simulink model "SimBG"  (R2023b)
settings: Solver=VariableStepAuto  StartTime=0.0  StopTime=t_sim  MaxStep=1e-2  RelTol=1e-3
values from neighbouring files (symbols this model uses):
  BG_0 = 120    [Batch_test_Cryer.m]    (also in Step_test.m; example_batch_testing.m; glucagon_dependency_test.m; init.m)
  control_flag = false    [Batch_test_Cryer.m]    (also in example_batch_testing.m; glucagon_dependency_test.m; init.m)
  G_GNG = 6    [Batch_test_Cryer.m]    (also in example_batch_testing.m; glucagon_dependency_test.m; init.m)
  glucagon_dose = 1e7    (= 10000000)    [Batch_test_Cryer.m]    (also in example_batch_testing.m; glucagon_dependency_test.m; init.m)
  Hyper_Hyst_H = (Hyper_Threshold + 10)/18    (= 10.5555555556)    [Batch_test_Cryer.m]    (also in example_batch_testing.m; glucagon_dependency_test.m; init.m)
  Hyper_Hyst_L = (Hyper_Threshold - 10)/18    (= 9.44444444444)    [Batch_test_Cryer.m]    (also in example_batch_testing.m; glucagon_dependency_test.m; init.m)
  Hyper_Threshold = 180    [Batch_test_Cryer.m]    (also in example_batch_testing.m; glucagon_dependency_test.m; init.m)
  Hypo_Hyst_H = (Hypo_Threshold+10)/18    (= 4.44444444444)    [Batch_test_Cryer.m]    (also in example_batch_testing.m; glucagon_dependency_test.m; init.m)
  Hypo_Hyst_L = (Hypo_Threshold-10)/18    (= 3.33333333333)    [Batch_test_Cryer.m]    (also in example_batch_testing.m; glucagon_dependency_test.m; init.m)
  Hypo_Threshold = 70    [Batch_test_Cryer.m]    (also in example_batch_testing.m; glucagon_dependency_test.m; init.m)
  k_bi = rand*0.05+0.075    [Batch_test_Cryer.m]    (also in example_batch_testing.m; init.m)
  K_d_glu = 2.484    [Batch_test_Cryer.m]    (also in example_batch_testing.m; glucagon_dependency_test.m; init.m = 1)
  K_d_ins = 379.0122/ICR -5.8677    [Batch_test_Cryer.m]    (also in example_batch_testing.m; glucagon_dependency_test.m; init.m)
  K_i_glu = 0    [Batch_test_Cryer.m]    (also in example_batch_testing.m; glucagon_dependency_test.m; init.m)
  K_i_ins = 0    [Batch_test_Cryer.m]    (also in example_batch_testing.m; glucagon_dependency_test.m; init.m)
  K_p_glu = 0.10976    [Batch_test_Cryer.m]    (also in example_batch_testing.m; glucagon_dependency_test.m; init.m = 0.1)
  K_p_ins = 0.1    [Batch_test_Cryer.m]    (also in example_batch_testing.m; glucagon_dependency_test.m; init.m)
  M_g = 180.16    [Batch_test_Cryer.m]    (also in example_batch_testing.m; glucagon_dependency_test.m; init.m)
  sig_n = 10    [Batch_test_Cryer.m]    (also in example_batch_testing.m; glucagon_dependency_test.m; init.m)
  T_CGM = 5    [Batch_test_Cryer.m]    (also in example_batch_testing.m; glucagon_dependency_test.m; init.m)
  T_CTRL = 5    [Batch_test_Cryer.m]    (also in example_batch_testing.m; glucagon_dependency_test.m; init.m)
  t_sim = minutes(end_time - start_time)    [Batch_test_Cryer.m]    (also in Step_test.m = 1800; example_batch_testing.m; glucagon_dependency_test.m; init.m = 1800)
  TDD_limit = 0.6*W*1000    (= 42000)    [Batch_test_Cryer.m]    (also in example_batch_testing.m; glucagon_dependency_test.m; init.m)
  U_b0 = fzero(f, 10)    [Batch_test_Cryer.m]    (also in Step_test.m; cohort_generation.m; example_batch_testing.m; glucagon_dependency_test.m)
  W = 70    [Batch_test_Cryer.m]    (also in example_batch_testing.m; glucagon_dependency_test.m; init.m)
undefined symbols (not defined in the file or in its folder): A_G, C_b, C_E50, CL_FC, E_max, F_01, fc1_bias, fc1_weight, fc2_bias, fc2_weight, gru_bias_hh_l0, gru_bias_ih_l0, gru_weight_hh_l0, gru_weight_ih_l0, k_1, k_12, k_2, k_a1, k_a2, k_a3, k_e, S_D, S_E, S_T, t_max_G, t_max_I, V_G, V_I
libraries: simulink x1
settings Model: Creator=AnyuSHAN  LastModifiedBy=djcry

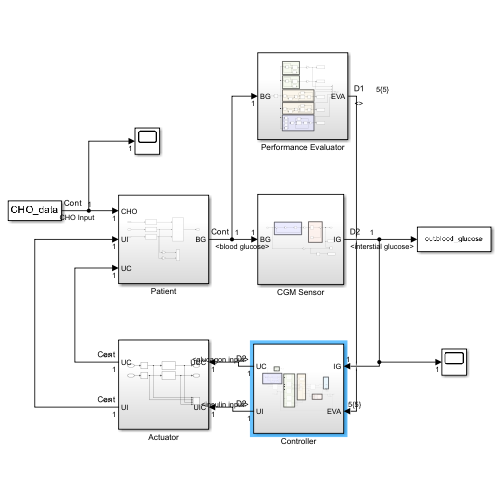
[thumbnail: Simulink's stored preview of the top-level diagram]
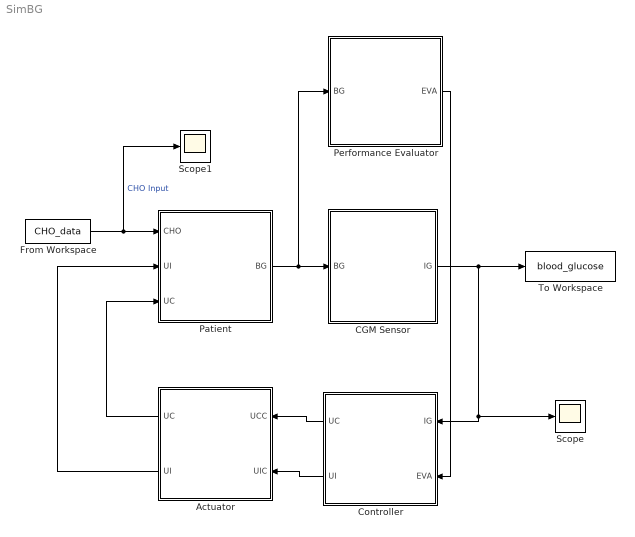
== system SimBG ==
  Actuator : Subsystem
  CGM Sensor : Subsystem
  Controller : Subsystem
  From Workspace : FromWorkspace  VariableName=CHO_data
  Patient : Subsystem
  Performance Evaluator : Subsystem
  Scope : Scope
  Scope1 : Scope
  To Workspace : ToWorkspace  VariableName=blood_glucose  SaveFormat=Timeseries  SampleTime=-1
  wires:
  From Workspace/1 -> Scope1/1, Patient/1(CHO)  "CHO Input"
  Patient/1(BG) -> Performance Evaluator/1(BG), CGM Sensor/1(BG)
  CGM Sensor/1(IG) -> Scope/1, Controller/1(IG), To Workspace/1
  Actuator/1(UC) -> Patient/3(UC)
  Actuator/2(UI) -> Patient/2(UI)
  Controller/1(UC) -> Actuator/1(UCC)
  Controller/2(UI) -> Actuator/2(UIC)
  Performance Evaluator/1(EVA) -> Controller/2(EVA)

== system SimBG/Actuator ==
  UCC : Inport
  UIC : Inport  Port=2
  Saturation : Saturate  UpperLimit=inf  LowerLimit=0
  Saturation1 : Saturate  UpperLimit=60000  LowerLimit=0
  Scope : Scope  NumInputPorts=4
  Transfer Fcn : TransferFcn  Denominator=[1]
  Transfer Fcn1 : TransferFcn  Denominator=[1]
  UC : Outport
  UI : Outport  Port=2
  wires:
  UCC/1 -> Saturation/1
  UIC/1 -> Saturation1/1
  Transfer Fcn/1 -> Scope/3, UC/1
  Transfer Fcn1/1 -> Scope/4, UI/1
  Saturation/1 -> Scope/1, Transfer Fcn/1
  Saturation1/1 -> Scope/2, Transfer Fcn1/1

== system SimBG/CGM Sensor ==
  note: Non-ideal Sensor
  note: Blood-Glucose to Interstitial-Glucose Delay
  BG : Inport
  Band-Limited White Noise : simulink/Sources/Band-Limited White Noise  Cov=[sig_n^2]  Ts=5  seed=[23341]
  Gain : Gain  Gain=k_bi
  Gain2 : Gain  Gain=18
  Integrator : Integrator  InitialCondition=BG_0/18
  Sampling Rate : RateTransition  InitialCondition=BG_0  OutPortSampleTime=T_CGM
  Sampling Rate1 : RateTransition  InitialCondition=BG_0  OutPortSampleTime=T_CGM
  Scope : Scope  NumInputPorts=2
  Sum : Sum  Inputs=|+-
  Sum1 : Sum  Inputs=|++
  To Workspace : ToWorkspace  VariableName=real_bg  SaveFormat=Timeseries  SampleTime=-1
  To Workspace1 : ToWorkspace  VariableName=CGM  SaveFormat=Timeseries  SampleTime=-1
  Unit Conversion : Gain  Gain=18
  IG : Outport
  wires:
  BG/1 -> Gain2/1, Sum/1
  Sum/1 -> Gain/1
  Gain/1 -> Integrator/1
  Integrator/1 -> Unit Conversion/1, Sum/2
  Band-Limited White Noise/1 -> Sum1/2  "Sensor Noise"
  Unit Conversion/1 -> Sampling Rate/1
  Gain2/1 -> Sampling Rate1/1, Scope/2  "blood glucose"
  Sampling Rate/1 -> Sum1/1
  Sum1/1 -> To Workspace1/1, Scope/1, IG/1  "interstial glucose"
  Sampling Rate1/1 -> To Workspace/1

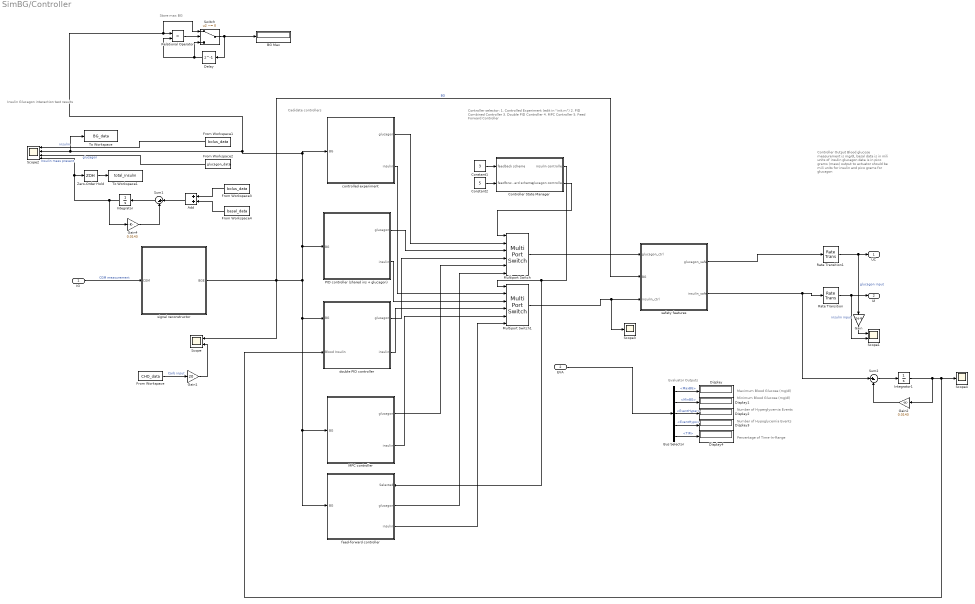
== system SimBG/Controller ==
  note: Insulin Glucagon interaction test results
  note: Controller Output
      |
      | Blood glucose measurement is
      | mg/dL basal data is in mili units
      | of insulin glucagon data is in pico
      | grams (mass)
      |
      | output to actuator should be mili
      | units for insulin and pico grams
      | for glucagon
  note: Evaluator Outputs
  note: Maximum Blood Glucose (mg/dl)
  note: Minimum Blood Glucose (mg/dl)
  note: Number of Hyperglycemia Events
  note: Number of Hypoglycemia Events
  note: Percentage of Time-In-Range
  note: Cadidate controllers
  note: Controller selector:
      |
      |     1. Controlled Experiment (edit in "init.m")
      |     2. PID Combined Controller
      |     3. Double PID Controller
      |     4. MPC Controller
      |     5. Feed Forward Controller
  note: Store max BG
  IG : Inport
  EVA : Inport  Port=2
  Add : Sum
  "BG Max " : Display
  Bus Selector : BusSelector  OutputSignals=MaxBG,MinBG,EventHyper,EventHypo,TIR
  Constant1 : Constant  Value=3
  Constant2 : Constant  Value=5
  Controller State Manager : Subsystem
  Delay : Delay  DelayLength=1
  Display{,1..4} (5 alike) : Display
  From Workspace : FromWorkspace  VariableName=CHO_data
  From Workspace1 : FromWorkspace  VariableName=bolus_data
  From Workspace2 : FromWorkspace  VariableName=glucagon_data
  From Workspace3 : FromWorkspace  VariableName=bolus_data
  From Workspace4 : FromWorkspace  VariableName=basal_data
  Gain : Gain  Gain=1e-6
  Gain1 : Gain  Gain=20
  Gain2 : Gain  Gain=0.0143
  Gain4 : Gain  Gain=0.0143
  Integrator : Integrator
  Integrator1 : Integrator
  MPC controller : Subsystem
  Multiport Switch : MultiPortSwitch  Inputs=5  SaturateOnIntegerOverflow=off  InputSameDT=off
  Multiport Switch1 : MultiPortSwitch  Inputs=5  SaturateOnIntegerOverflow=off  InputSameDT=off
  "PID controller (shared ins + glucagon) " : Subsystem
  Rate Transition : RateTransition  OutPortSampleTime=T_CTRL
  Rate Transition1 : RateTransition  OutPortSampleTime=T_CTRL
  Relational Operator : RelationalOperator  Operator=>  OutDataTypeStr=boolean  RndMeth=Simplest  InputSameDT=off
  Scope : Scope  NumInputPorts=2
  Scope1 : Scope  NumInputPorts=2
  Scope2 : Scope  NumInputPorts=4
  Scope3 : Scope
  Scope4 : Scope
  Sum1 : Sum  Inputs=|+-
  Sum2 : Sum  Inputs=|+-
  Switch : Switch  Criteria=u2 ~= 0  SaturateOnIntegerOverflow=off  InputSameDT=off
  To Workspace : ToWorkspace  VariableName=BG_data  SampleTime=-1
  To Workspace1 : ToWorkspace  VariableName=total_insulin  SampleTime=-1
  Zero-Order Hold : ZeroOrderHold  SampleTime=T_CGM
  controlled experiment : Subsystem
  "double PID controller " : Subsystem
  feed-forward controller : Subsystem
      settings: PortSchema="{\"entries\":[{\"content\":{\"sides\":[{\"content\":{\"connectorIds\":[\"In1\"]},\"type\":\"ConnectorPlacement.EquallySpacedRectSide\",\"uuid\":\"dbaf1568-f06b-4b59-a78d-fcd88c99f30c\"},{\"content\":{\"connectorIds\":[\"In2\",\"Out1\",\"Out2\"],\"side\":\"RIGHT\"},\"type\":\"ConnectorPlacement.EquallySpacedRectSide\",\"uuid\":\"a5934e92-00f4-4f02-9cc0-b5d8731ec04b\"},{\"content\":{\"side\":\"TOP\"},\"type\":\"ConnectorPlacement.EquallySpacedRectSide\",\"uuid\":\"d354fd2d-5aba-4440-830b-950c4e2ceeab\"}]},\"type\":\"ConnectorPlacement.EquallySpacedConnector\",\"uuid\":\"501b8066-4d36-4767-bbbc-30e356c73da4\"}],\"packageUris\":[\"http://schema.mathworks.com/mf0/Connector/R2020b\"],\"version\":\"1.0\"}"
  safety features : Subsystem
  signal reconstructor : Subsystem
  UC : Outport
  UI : Outport  Port=2
  wires:
  Rate Transition/1 -> Scope1/2, UI/1  "insulin input"
  Rate Transition1/1 -> UC/1, Gain/1  "glucagon input"
  EVA/1 -> Bus Selector/1
  Bus Selector/1 -> Display/1  "<MaxBG>"
  Bus Selector/2 -> Display1/1  "<MinBG>"
  Bus Selector/3 -> Display2/1  "<EventHyper>"
  Bus Selector/4 -> Display3/1  "<EventHypo>"
  Bus Selector/5 -> Display4/1  "<TIR>"
  safety features/1(glucagon_safe) -> Rate Transition1/1
  Gain/1 -> Scope1/1
  safety features/2(insulin_safe) -> Sum2/1, Rate Transition/1
  From Workspace/1 -> Gain1/1  "Carb input"
  Controller State Manager/1(insulin controller) -> feed-forward controller/2(Selected), Multiport Switch1/1
  MPC controller/2(insulin) -> Multiport Switch1/5
  Controller State Manager/2(glucagon controller) -> Multiport Switch/1
  "double PID controller "/1(glucagon) -> Multiport Switch/4
  IG/1 -> signal reconstructor/1(CGM)  "CGM measurement"
  "double PID controller "/2(insulin) -> Multiport Switch1/4
  Multiport Switch1/1 -> Scope3/1, safety features/3(insulin_ctrl)
  feed-forward controller/1(glucagon) -> Multiport Switch/6
  controlled experiment/2(insulin) -> Multiport Switch1/2
  controlled experiment/1(glucagon) -> Multiport Switch/2
  "PID controller (shared ins + glucagon) "/2(insulin) -> Multiport Switch1/3
  signal reconstructor/1(BGE) -> safety features/2(BG), Scope/1, controlled experiment/1(BG), Relational Operator/1, Switch/1, To Workspace/1, Scope2/2, "PID controller (shared ins + glucagon) "/1(BG), MPC controller/1(BG), feed-forward controller/1(BG), "double PID controller "/1(BG)  "BG"
  feed-forward controller/2(insulin) -> Multiport Switch1/6
  "PID controller (shared ins + glucagon) "/1(glucagon) -> Multiport Switch/3
  Constant2/1 -> Controller State Manager/2(feedforward scheme)
  Multiport Switch/1 -> safety features/1(glucagon_ctrl)
  MPC controller/1(glucagon) -> Multiport Switch/5
  Constant1/1 -> Controller State Manager/1(feedback scheme)
  Gain1/1 -> Scope/2
  From Workspace2/1 -> Scope2/3  "glucagon"
  From Workspace1/1 -> Scope2/1  "insulin"
  Switch/1 -> "BG Max "/1, Delay/1
  Delay/1 -> Relational Operator/2, Switch/3
  Relational Operator/1 -> Switch/2
  From Workspace3/1 -> Add/1
  From Workspace4/1 -> Add/2
  Add/1 -> Sum1/1
  Sum1/1 -> Integrator/1
  Integrator/1 -> Scope2/4, Zero-Order Hold/1, Gain4/1  "Insulin mass present"
  Gain4/1 -> Sum1/2
  Zero-Order Hold/1 -> To Workspace1/1
  Gain2/1 -> Sum2/2
  Integrator1/1 -> "double PID controller "/2(Blood Insulin), Scope4/1, Gain2/1
  Sum2/1 -> Integrator1/1

== system SimBG/Patient ==
  CHO : Inport
  UI : Inport  Port=2
  UC : Inport  Port=3
  Gain : Gain  Gain=1/C_b
  Gain1 : Gain  Gain=(k_e*V_I*W)/U_b0
  Glucagon PK : Subsystem
  Glucose PD : Subsystem
  Gut Absorption : Subsystem
  Insulin PK : Subsystem
  Scope : Scope  NumInputPorts=2
  BG : Outport
  wires:
  UI/1 -> Insulin PK/1(UI)
  UC/1 -> Glucagon PK/1(UC)
  CHO/1 -> Gut Absorption/1(CHO)
  Insulin PK/1(I) -> Gain1/1, Glucose PD/2(I)
  Gut Absorption/1(U) -> Glucose PD/1(U)
  Glucose PD/1(BG) -> BG/1
  Glucagon PK/1(C) -> Gain/1, Glucose PD/3(C)
  Gain1/1 -> Scope/1  "insulin relative"
  Gain/1 -> Scope/2  "glucagon relative"

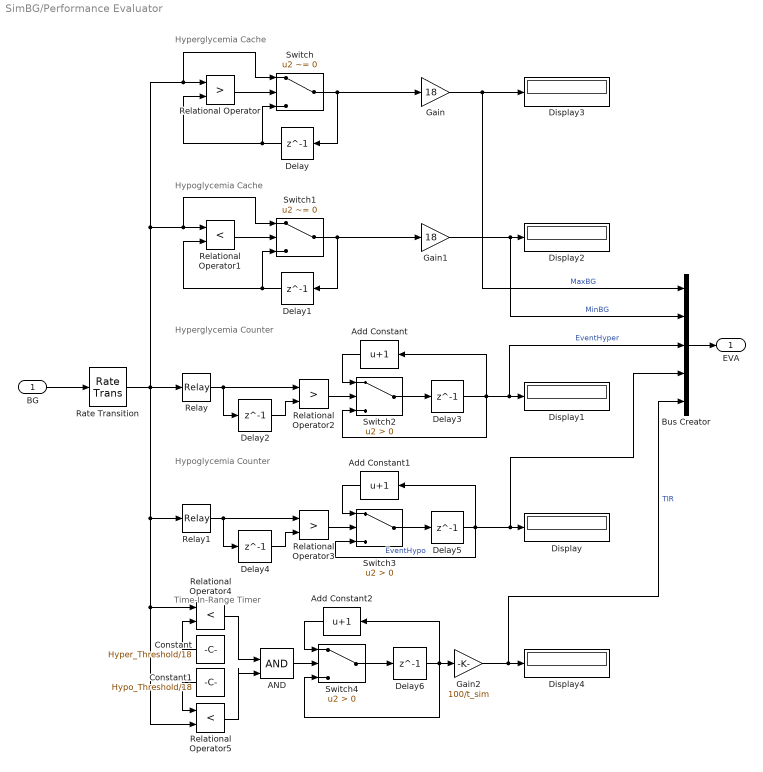
== system SimBG/Performance Evaluator ==
  note: Time-In-Range Timer
  note: Hyperglycemia Counter
  note: Hypoglycemia Cache
  note: Hyperglycemia Cache
  note: Hypoglycemia Counter
  BG : Inport
  AND : Logic  IconShape=distinctive  AllPortsSameDT=off  OutDataTypeStr=boolean
  Add Constant : Bias  Bias=1  SaturateOnIntegerOverflow=off
  Add Constant1 : Bias  Bias=1  SaturateOnIntegerOverflow=off
  Add Constant2 : Bias  Bias=1  SaturateOnIntegerOverflow=off
  Bus Creator : BusCreator  Inputs=5
  Constant : Constant  Value=Hyper_Threshold/18
  Constant1 : Constant  Value=Hypo_Threshold/18
  Delay{,2..6} (6 alike) : Delay  DelayLength=1
  Delay1 : Delay  DelayLength=1  InitialCondition=100
  Display{,1..4} (5 alike) : Display
  Gain : Gain  Gain=18
  Gain1 : Gain  Gain=18
  Gain2 : Gain  Gain=100/t_sim
  Rate Transition : RateTransition  OutPortSampleTime=1
  Relational Operator : RelationalOperator  Operator=>  OutDataTypeStr=boolean  RndMeth=Simplest  InputSameDT=off
  Relational Operator1 : RelationalOperator  Operator=<  OutDataTypeStr=boolean  RndMeth=Simplest  InputSameDT=off
  Relational Operator2 : RelationalOperator  Operator=>  OutDataTypeStr=boolean  RndMeth=Simplest  InputSameDT=off
  Relational Operator3 : RelationalOperator  Operator=>  OutDataTypeStr=boolean  RndMeth=Simplest  InputSameDT=off
  Relational Operator4 : RelationalOperator  Operator=<  OutDataTypeStr=boolean  RndMeth=Simplest  InputSameDT=off
  Relational Operator5 : RelationalOperator  Operator=<  OutDataTypeStr=boolean  RndMeth=Simplest  InputSameDT=off
  Relay : Relay  OnSwitchValue=Hyper_Hyst_H  OffSwitchValue=Hyper_Hyst_L
  Relay1 : Relay  OnSwitchValue=Hypo_Hyst_H  OffSwitchValue=Hypo_Hyst_L  OnOutputValue=0  OffOutputValue=1
  Switch : Switch  Criteria=u2 ~= 0  SaturateOnIntegerOverflow=off  InputSameDT=off
  Switch1 : Switch  Criteria=u2 ~= 0  SaturateOnIntegerOverflow=off  InputSameDT=off
  Switch2 : Switch  Criteria=u2 > Threshold  SaturateOnIntegerOverflow=off  InputSameDT=off
  Switch3 : Switch  Criteria=u2 > Threshold  SaturateOnIntegerOverflow=off  InputSameDT=off
  Switch4 : Switch  Criteria=u2 > Threshold  SaturateOnIntegerOverflow=off  InputSameDT=off
  EVA : Outport
  wires:
  Relational Operator/1 -> Switch/2
  Switch/1 -> Gain/1, Delay/1
  Delay/1 -> Relational Operator/2, Switch/3
  BG/1 -> Rate Transition/1
  Relational Operator1/1 -> Switch1/2
  Delay1/1 -> Relational Operator1/2, Switch1/3
  Switch1/1 -> Gain1/1, Delay1/1
  Relay/1 -> Relational Operator2/1, Delay2/1
  Delay2/1 -> Relational Operator2/2
  Relational Operator2/1 -> Switch2/2
  Switch2/1 -> Delay3/1
  Delay3/1 -> Bus Creator/3, Display1/1, Add Constant/1, Switch2/3  "EventHyper"
  Add Constant/1 -> Switch2/1
  Delay4/1 -> Relational Operator3/2
  Rate Transition/1 -> Switch/1, Relational Operator/1, Switch1/1, Relational Operator1/1, Relational Operator5/2, Relational Operator4/1, Relay1/1, Relay/1
  Relational Operator3/1 -> Switch3/2
  Delay5/1 -> Bus Creator/4, Display/1, Switch3/3, Add Constant1/1  "EventHypo"
  Add Constant1/1 -> Switch3/1
  Relay1/1 -> Relational Operator3/1, Delay4/1
  Switch3/1 -> Delay5/1
  Gain/1 -> Bus Creator/1, Display3/1  "MaxBG"
  Gain1/1 -> Bus Creator/2, Display2/1  "MinBG"
  Constant/1 -> Relational Operator4/2
  Constant1/1 -> Relational Operator5/1
  Relational Operator4/1 -> AND/1
  Relational Operator5/1 -> AND/2
  Add Constant2/1 -> Switch4/1
  Switch4/1 -> Delay6/1
  Delay6/1 -> Add Constant2/1, Gain2/1, Switch4/3
  AND/1 -> Switch4/2
  Gain2/1 -> Bus Creator/5, Display4/1  "TIR"
  Bus Creator/1 -> EVA/1

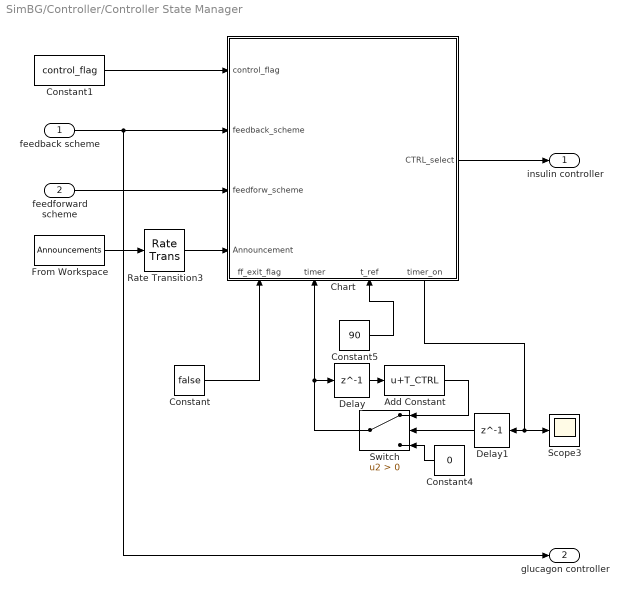
== system SimBG/Controller/Controller State Manager ==
  feedback scheme : Inport
  feedforward scheme : Inport  Port=2
  Add Constant : Bias  Bias=T_CTRL  SaturateOnIntegerOverflow=off
  Chart : Stateflow chart  TreatAsAtomicUnit=on
      settings: PortSchema="{\"entries\":[{\"content\":{\"sides\":[{\"content\":{\"connectorIds\":[\"In6\",\"In4\",\"In5\",\"In7\"]},\"type\":\"ConnectorPlacement.EquallySpacedRectSide\",\"uuid\":\"e6899742-d930-4cdd-9e73-f4511c9292a8\"},{\"content\":{\"connectorIds\":[\"Out2\"],\"side\":\"RIGHT\"},\"type\":\"ConnectorPlacement.EquallySpacedRectSide\",\"uuid\":\"ec367191-0ded-4e49-940d-e1c38365304e\"},{\"content\":{\"side\":\"TOP\"},\"type\":\"ConnectorPlacement.EquallySpacedRectSide\",\"uuid\":\"36bc0aba-d7ee-40bb-abeb-760521564d0e\"},{\"content\":{\"connectorIds\":[\"In3\",\"In1\",\"In2\",\"Out1\"],\"side\":\"BOTTOM\"},\"type\":\"ConnectorPlacement.EquallySpacedRectSide\",\"uuid\":\"328131cb-e716-44f1-bdd5-5ff70ee895ba\"}]},\"type\":\"ConnectorPlacement.EquallySpacedConnector\",\"uuid\":\"b766fa1d-d143-42bc-8f8c-60374aa390c3\"}],\"packageUris\":[\"http://schema.mathworks.com/mf0/Connector/R2020b\"],\"version\":\"1.0\"}"
  Constant : Constant  Value=false
  Constant1 : Constant  Value=control_flag
  Constant4 : Constant  Value=0
  Constant5 : Constant  Value=90
  Delay : Delay  DelayLength=1
  Delay1 : Delay  DelayLength=1
  From Workspace : FromWorkspace  VariableName=Announcements
  Rate Transition3 : RateTransition  OutPortSampleTime=T_CTRL
  Scope3 : Scope
  Switch : Switch  Criteria=u2 > Threshold  SaturateOnIntegerOverflow=off  InputSameDT=off
  insulin controller : Outport
  glucagon controller : Outport  Port=2
  wires:
  Chart/2(CTRL_select) -> insulin controller/1
  Rate Transition3/1 -> Chart/7(Announcement)
  Chart/1(timer_on) -> Scope3/1, Delay1/1
  Add Constant/1 -> Switch/1
  feedback scheme/1 -> Chart/4(feedback_scheme), glucagon controller/1
  Constant4/1 -> Switch/3
  feedforward scheme/1 -> Chart/5(feedforw_scheme)
  Constant5/1 -> Chart/2(t_ref)
  Switch/1 -> Delay/1, Chart/1(timer)
  From Workspace/1 -> Rate Transition3/1
  Constant1/1 -> Chart/6(control_flag)
  Delay/1 -> Add Constant/1
  Delay1/1 -> Switch/2
  Constant/1 -> Chart/3(ff_exit_flag)

== system SimBG/Controller/MPC controller ==
  BG : Inport
  Demux : Demux  Outputs=2
  MPC Function : MATLAB Function  TreatAsAtomicUnit=on
  glucagon : Outport
  insulin : Outport  Port=2
  wires:
  MPC Function/1(u) -> Demux/1
  BG/1 -> MPC Function/1(y)
  Demux/1 -> insulin/1
  Demux/2 -> glucagon/1

== system SimBG/Controller/PID controller (shared ins + glucagon)  ==
  BG : Inport
  Constant2 : Constant  Value=0
  From Workspace : FromWorkspace  VariableName=CHO_data
  Gain1 : Gain  Gain=-glucagon_dose
  Gain2 : Gain  Gain=20
  Saturation1 : Saturate  UpperLimit=inf  LowerLimit=0
  Scope : Scope  NumInputPorts=9
  "Standard PID controller " : Subsystem
  Switch1 : Switch  Criteria=u2 > Threshold  Threshold=-16  SaturateOnIntegerOverflow=off  InputSameDT=off
  glucagon : Outport
  insulin : Outport  Port=2
  wires:
  "Standard PID controller "/4(Out4) -> Scope/7
  "Standard PID controller "/1(controller ouput) -> Saturation1/1, Switch1/3, Switch1/2, Scope/4
  "Standard PID controller "/2(Out2) -> Scope/5
  Saturation1/1 -> insulin/1, Scope/1  "insulin"
  Switch1/1 -> Scope/2, Gain1/1  "glucagon"
  BG/1 -> Scope/9, "Standard PID controller "/1(Estimated BG (mg/dL))
  Gain1/1 -> glucagon/1  "glucagon"
  Constant2/1 -> Switch1/1
  Gain2/1 -> Scope/8  "20 * carb input"
  From Workspace/1 -> Gain2/1  "Carb input"
  "Standard PID controller "/3(Out1) -> Scope/6

== system SimBG/Controller/controlled experiment ==
  BG : Inport
  From Workspace : FromWorkspace  VariableName=glucagon_data
  From Workspace2 : FromWorkspace  VariableName=bolus_data
  Terminator : Terminator
  glucagon : Outport
  insulin : Outport  Port=2
  wires:
  From Workspace2/1 -> insulin/1
  From Workspace/1 -> glucagon/1
  BG/1 -> Terminator/1

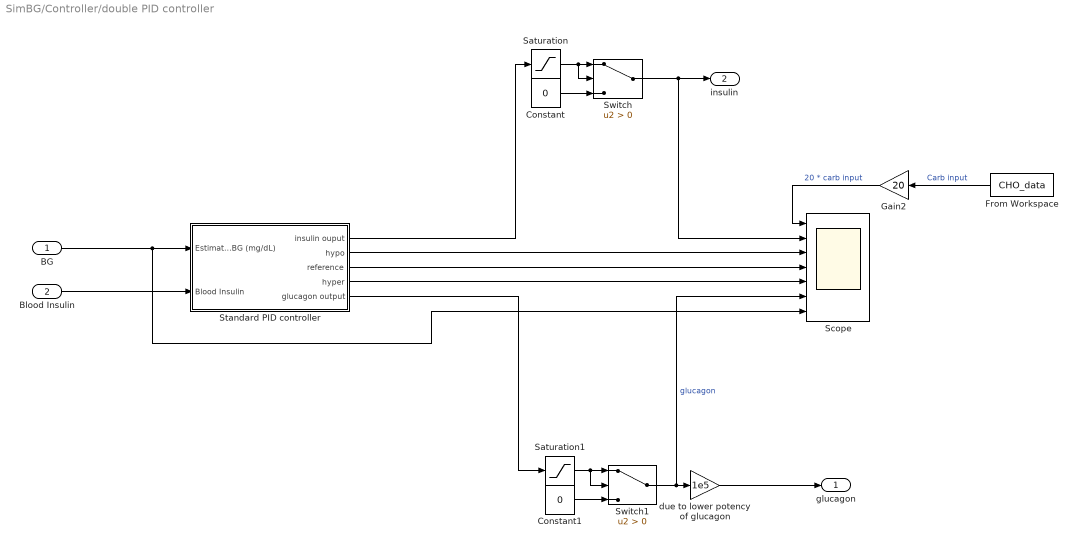
== system SimBG/Controller/double PID controller  ==
  BG : Inport
  Blood Insulin : Inport  Port=2
  Constant : Constant  Value=0
  Constant1 : Constant  Value=0
  From Workspace : FromWorkspace  VariableName=CHO_data
  Gain2 : Gain  Gain=20
  Saturation : Saturate  UpperLimit=inf  LowerLimit=0
  Saturation1 : Saturate  UpperLimit=inf  LowerLimit=0
  Scope : Scope  NumInputPorts=7
  "Standard PID controller " : Subsystem
  Switch : Switch  Criteria=u2 > Threshold  SaturateOnIntegerOverflow=off  InputSameDT=off
  Switch1 : Switch  Criteria=u2 > Threshold  SaturateOnIntegerOverflow=off  InputSameDT=off
  due to lower potency of glucagon : Gain  Gain=1e5
  glucagon : Outport
  insulin : Outport  Port=2
  wires:
  BG/1 -> Scope/7, "Standard PID controller "/1(Estimated BG (mg/dL))
  "Standard PID controller "/1(insulin ouput) -> Saturation/1
  "Standard PID controller "/2(hypo) -> Scope/3
  "Standard PID controller "/3(reference) -> Scope/4
  "Standard PID controller "/4(hyper) -> Scope/5
  "Standard PID controller "/5(glucagon output) -> Saturation1/1
  Gain2/1 -> Scope/1  "20 * carb input"
  From Workspace/1 -> Gain2/1  "Carb input"
  Saturation/1 -> Switch/2, Switch/1
  Constant/1 -> Switch/3
  Switch/1 -> insulin/1, Scope/2
  Saturation1/1 -> Switch1/2, Switch1/1
  Constant1/1 -> Switch1/3
  Switch1/1 -> Scope/6, due to lower potency of glucagon/1  "glucagon"
  due to lower potency of glucagon/1 -> glucagon/1
  Blood Insulin/1 -> "Standard PID controller "/2(Blood Insulin)

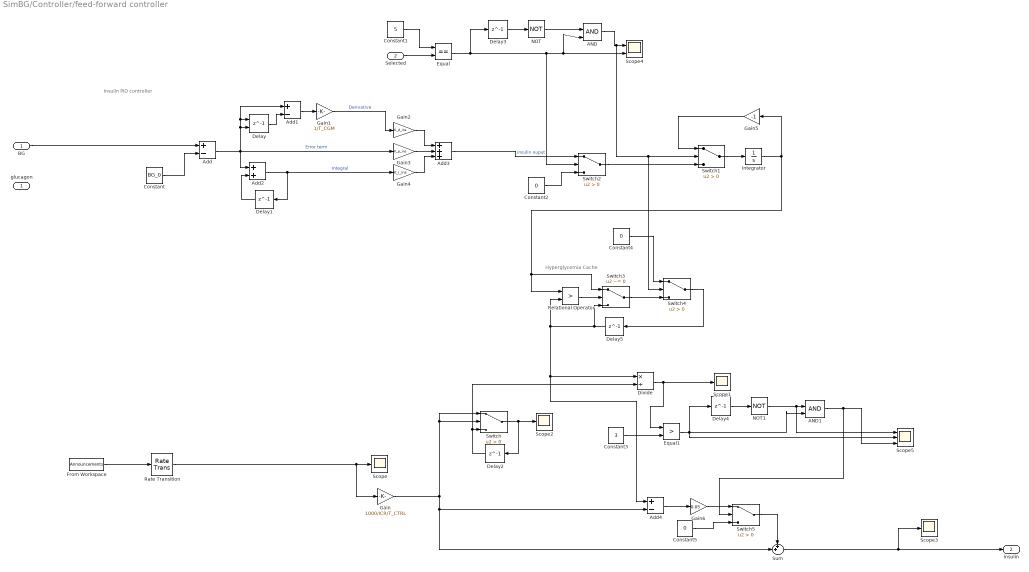
== system SimBG/Controller/feed-forward controller ==
  note: Insulin PID controller
  note: Hyperglycemia Cache
  BG : Inport
  Selected : Inport  Port=2
  AND : Logic  IconShape=distinctive  AllPortsSameDT=off  OutDataTypeStr=boolean
  AND1 : Logic  IconShape=distinctive  AllPortsSameDT=off  OutDataTypeStr=boolean
  Add : Sum  Inputs=+-
  Add1 : Sum  Inputs=+-
  Add2 : Sum
  Add3 : Sum  Inputs=+++
  Add4 : Sum  Inputs=+-
  Constant : Constant  Value=BG_0
  Constant1 : Constant  Value=5
  Constant2 : Constant  Value=0
  Constant3 : Constant  Value=3
  Constant4 : Constant  Value=0
  Constant5 : Constant  Value=0
  Delay : Delay  DelayLength=1  InitialConditionSource=Input port
      settings: InputPortMap=u0,p4
  Delay{1..5} (5 alike) : Delay  DelayLength=1
  Divide : Product  Inputs=*/
  Equal : RelationalOperator  Operator===  OutDataTypeStr=boolean  RndMeth=Simplest  InputSameDT=off
  Equal1 : RelationalOperator  Operator=>  OutDataTypeStr=boolean  RndMeth=Simplest  InputSameDT=off
  From Workspace : FromWorkspace  VariableName=Announcements
  Gain : Gain  Gain=1000/ICR/T_CTRL
  Gain1 : Gain  Gain=1/T_CGM
  Gain2 : Gain  Gain=K_d_ins
  Gain3 : Gain  Gain=K_p_ins
  Gain4 : Gain  Gain=K_i_ins
  Gain5 : Gain  Gain=-1
  Gain6 : Gain  Gain=0.05
  Integrator : Integrator
  NOT : Logic  Operator=NOT  IconShape=distinctive  AllPortsSameDT=off  OutDataTypeStr=boolean
  NOT1 : Logic  Operator=NOT  IconShape=distinctive  AllPortsSameDT=off  OutDataTypeStr=boolean
  Rate Transition : RateTransition  OutPortSampleTime=T_CTRL
  Relational Operator : RelationalOperator  Operator=>  OutDataTypeStr=boolean  RndMeth=Simplest  InputSameDT=off
  Scope{,1..3} (4 alike) : Scope
  Scope4 : Scope  NumInputPorts=2
  Scope5 : Scope  NumInputPorts=3
  Sum : Sum  Inputs=++|
  Switch{,1..2,4..5} (5 alike) : Switch  Criteria=u2 > Threshold  SaturateOnIntegerOverflow=off  InputSameDT=off
  Switch3 : Switch  Criteria=u2 ~= 0  SaturateOnIntegerOverflow=off  InputSameDT=off
  glucagon : Outport
  insulin : Outport  Port=2
  wires:
  From Workspace/1 -> Rate Transition/1
  Rate Transition/1 -> Gain/1, Scope/1
  BG/1 -> Add/1
  Add/1 -> Add2/1, Delay/2, Delay/1, Add1/1, Gain3/1  "Error term"
  Delay1/1 -> Add2/2
  Gain2/1 -> Add3/1
  Add1/1 -> Gain1/1
  Gain3/1 -> Add3/2
  Add2/1 -> Gain4/1, Delay1/1  "Integral"
  Gain4/1 -> Add3/3
  Delay/1 -> Add1/2
  Constant/1 -> Add/2
  Gain1/1 -> Gain2/1  "Derivative"
  Switch1/1 -> Integrator/1
  Switch/1 -> Scope2/1, Delay2/1
  Delay2/1 -> Divide/2, Switch/3
  Gain5/1 -> Switch1/1
  Selected/1 -> Equal/2
  Constant1/1 -> Equal/1
  Equal/1 -> Delay3/1, AND/2, Scope4/2, Switch2/2
  Delay3/1 -> NOT/1
  NOT/1 -> AND/1
  AND/1 -> Switch4/2, Switch1/2, Scope4/1
  Switch2/1 -> Switch1/3
  Add3/1 -> Switch2/1  "insulin ouput"
  Constant2/1 -> Switch2/3
  Gain/1 -> Switch/2, Switch/1, Sum/2, Add4/2
  Sum/1 -> Scope3/1, insulin/1
  Divide/1 -> Equal1/1, Scope1/1
  NOT1/1 -> Scope5/1, AND1/1
  Delay4/1 -> NOT1/1
  Equal1/1 -> Scope5/2, Delay4/1, AND1/2
  Constant3/1 -> Equal1/2
  Delay5/1 -> Relational Operator/2, Add4/1, Divide/1, Switch3/3
  Integrator/1 -> Gain5/1, Switch3/1, Relational Operator/1
  Relational Operator/1 -> Switch3/2
  Switch3/1 -> Switch4/3
  Switch4/1 -> Delay5/1
  Constant4/1 -> Switch4/1
  AND1/1 -> Switch5/2, Scope5/3
  Switch5/1 -> Sum/1
  Add4/1 -> Gain6/1
  Gain6/1 -> Switch5/1
  Constant5/1 -> Switch5/3

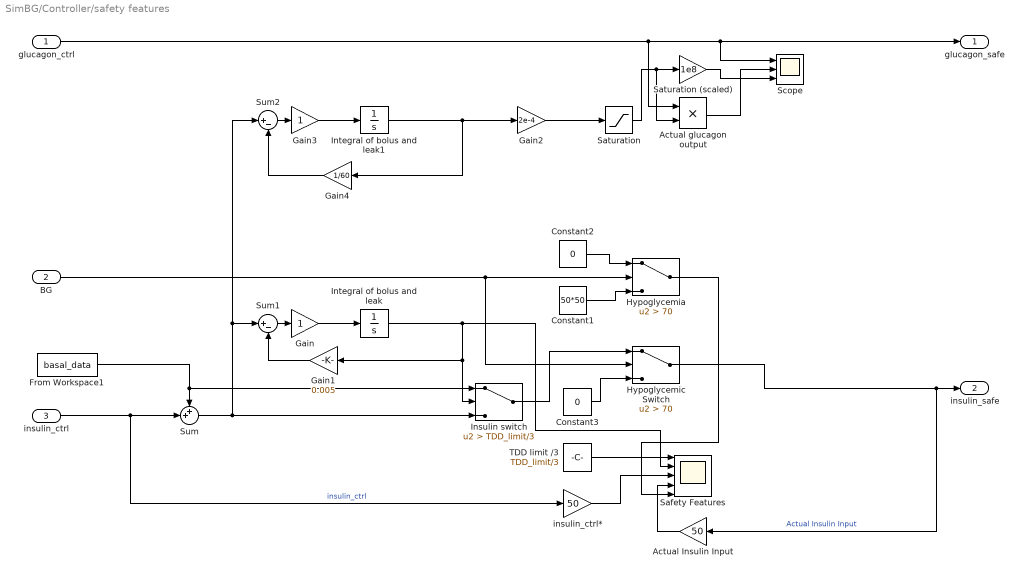
== system SimBG/Controller/safety features ==
  glucagon_ctrl : Inport
  BG : Inport  Port=2
  insulin_ctrl : Inport  Port=3
  Actual Insulin Input : Gain  Gain=50
  Actual glucagon output : Product  Inputs=**
  Constant1 : Constant  Value=50*50
  Constant2 : Constant  Value=0
  Constant3 : Constant  Value=0
  From Workspace1 : FromWorkspace  VariableName=basal_data
  Gain : Gain
  Gain1 : Gain  Gain=0.005
  Gain2 : Gain  Gain=2e-4
  Gain3 : Gain
  Gain4 : Gain  Gain=1/60
  Hypoglycemia : Switch  Criteria=u2 > Threshold  Threshold=70  SaturateOnIntegerOverflow=off  InputSameDT=off
  Hypoglycemic Switch : Switch  Criteria=u2 > Threshold  Threshold=70  SaturateOnIntegerOverflow=off  InputSameDT=off
  Insulin switch : Switch  Criteria=u2 > Threshold  Threshold=TDD_limit/3  SaturateOnIntegerOverflow=off  InputSameDT=off
  Integral of bolus and leak : Integrator
  Integral of bolus and leak1 : Integrator
  Safety Features : Scope  NumInputPorts=5
  Saturation : Saturate  UpperLimit=1  LowerLimit=0
  Saturation (scaled) : Gain  Gain=1e8
  Scope : Scope  NumInputPorts=3
  Sum : Sum  Inputs=++|
  Sum1 : Sum  Inputs=|+-
  Sum2 : Sum  Inputs=|+-
  TDD limit /3 : Constant  Value=TDD_limit/3
  insulin_ctrl* : Gain  Gain=50
  glucagon_safe : Outport
  insulin_safe : Outport  Port=2
  wires:
  glucagon_ctrl/1 -> glucagon_safe/1, Scope/1, Actual glucagon output/1
  From Workspace1/1 -> Insulin switch/1, Sum/1
  Integral of bolus and leak/1 -> Insulin switch/2, Gain1/1, Safety Features/2
  BG/1 -> Hypoglycemia/2, Hypoglycemic Switch/2
  Insulin switch/1 -> Hypoglycemic Switch/1
  Hypoglycemic Switch/1 -> Actual Insulin Input/1, insulin_safe/1  "Actual Insulin Input"
  Constant3/1 -> Hypoglycemic Switch/3
  Sum1/1 -> Gain/1
  Gain1/1 -> Sum1/2
  Gain/1 -> Integral of bolus and leak/1
  insulin_ctrl/1 -> insulin_ctrl*/1, Sum/2  "insulin_ctrl"
  TDD limit /3/1 -> Safety Features/1
  Actual Insulin Input/1 -> Safety Features/4
  insulin_ctrl*/1 -> Safety Features/3
  Constant2/1 -> Hypoglycemia/1
  Constant1/1 -> Hypoglycemia/3
  Hypoglycemia/1 -> Safety Features/5
  Gain2/1 -> Saturation/1
  Saturation/1 -> Actual glucagon output/2, Saturation (scaled)/1
  Actual glucagon output/1 -> Scope/2
  Saturation (scaled)/1 -> Scope/3
  Gain3/1 -> Integral of bolus and leak1/1
  Integral of bolus and leak1/1 -> Gain2/1, Gain4/1
  Sum2/1 -> Gain3/1
  Sum/1 -> Sum2/1, Sum1/1, Insulin switch/3
  Gain4/1 -> Sum2/2

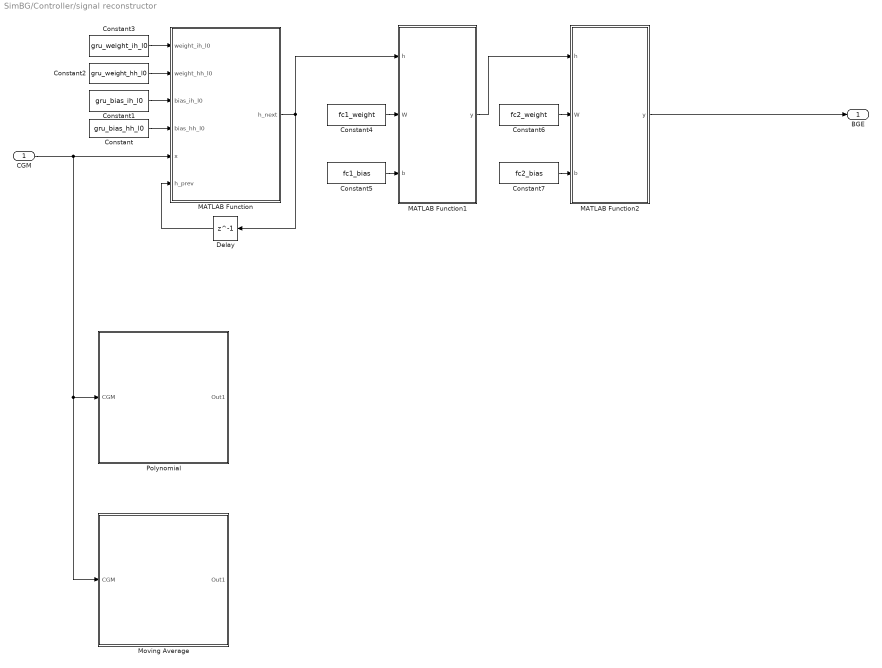
== system SimBG/Controller/signal reconstructor ==
  CGM : Inport  PortDimensions=1
  Constant : Constant  Value=gru_bias_hh_l0
  Constant1 : Constant  Value=gru_bias_ih_l0
  Constant2 : Constant  Value=gru_weight_hh_l0
  Constant3 : Constant  Value=gru_weight_ih_l0
  Constant4 : Constant  Value=fc1_weight
  Constant5 : Constant  Value=fc1_bias
  Constant6 : Constant  Value=fc2_weight
  Constant7 : Constant  Value=fc2_bias
  Delay : Delay  DelayLength=1  InitialCondition=zeros(length(gru_bias_hh_l0)/3, 1)
  MATLAB Function : MATLAB Function  TreatAsAtomicUnit=on
  MATLAB Function1 : MATLAB Function  TreatAsAtomicUnit=on
  MATLAB Function2 : MATLAB Function  TreatAsAtomicUnit=on
  Moving Average : Subsystem
  Polynomial : Subsystem
  BGE : Outport  PortDimensions=1
  wires:
  CGM/1 -> Moving Average/1(CGM), Polynomial/1(CGM), MATLAB Function/5(x)
  Constant/1 -> MATLAB Function/4(bias_hh_l0)
  Constant1/1 -> MATLAB Function/3(bias_ih_l0)
  Constant2/1 -> MATLAB Function/2(weight_hh_l0)
  Constant3/1 -> MATLAB Function/1(weight_ih_l0)
  MATLAB Function/1(h_next) -> MATLAB Function1/1(h), Delay/1
  Delay/1 -> MATLAB Function/6(h_prev)
  Constant4/1 -> MATLAB Function1/2(W)
  Constant5/1 -> MATLAB Function1/3(b)
  MATLAB Function1/1(y) -> MATLAB Function2/1(h)
  Constant7/1 -> MATLAB Function2/3(b)
  Constant6/1 -> MATLAB Function2/2(W)
  MATLAB Function2/1(y) -> BGE/1

== system SimBG/Patient/Glucagon PK ==
  note: Glucagon concentration in plasma
  note: Glucagon mass due to exogenous dosing, in plasma
  note: Glucagon mass due to exogenous dosing, in SC tissue
  UC : Inport
  Add Constant : Bias  Bias=C_b  SaturateOnIntegerOverflow=off
  Gain : Gain  Gain=k_1
  Gain1 : Gain  Gain=k_2
  Gain2 : Gain  Gain=1/(W*CL_FC)
  Integrator : Integrator  InitialCondition=C_b
  Integrator1 : Integrator  InitialCondition=C_b
  Sum : Sum  Inputs=-+|
  Sum1 : Sum  Inputs=-+|
  C : Outport
  wires:
  Integrator/1 -> Gain/1
  Gain1/1 -> Gain2/1, Sum1/1
  Gain/1 -> Sum1/2, Sum/1
  Integrator1/1 -> Gain1/1
  Sum/1 -> Integrator/1
  Sum1/1 -> Integrator1/1
  UC/1 -> Sum/2
  Gain2/1 -> Add Constant/1
  Add Constant/1 -> C/1  "Glucagon"

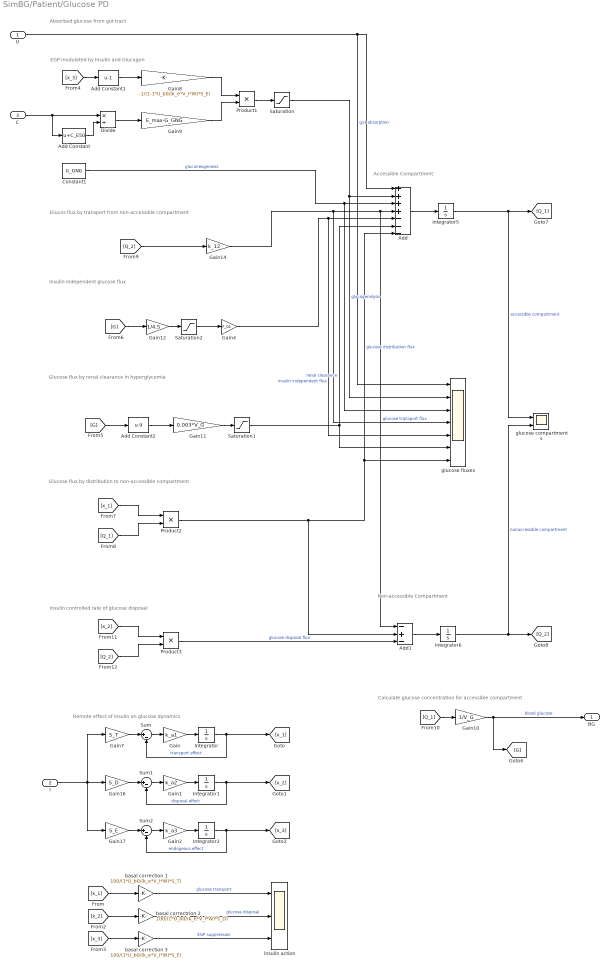
== system SimBG/Patient/Glucose PD ==
  note: Calculate glucose concentration for accessible compartment
  note: Non-accessible Compartment
  note: Accessible Compartment
  note: Insulin controlled rate of glucose disposal
  note: Absorbed glucose from gut tract
  note: Glucos flux by transport from non-accessible compartment
  note: Glucose flux by distribution to non-accessible compartment
  note: Insulin independent glucose flux
  note: Glucose flux by renal clearance in hyperglycemia
  note: EGP modulated by Insulin and Glucagon
  note: Remote effect of insulin on glucose dynamics
  U : Inport
  I : Inport  Port=2
  C : Inport  Port=3
  Add : Sum  Inputs=++++---
  Add Constant : Bias  Bias=C_E50  SaturateOnIntegerOverflow=off
  Add Constant1 : Bias  Bias=-1  SaturateOnIntegerOverflow=off
  Add Constant2 : Bias  Bias=-9  SaturateOnIntegerOverflow=off
  Add1 : Sum  Inputs=-+-
  Constant1 : Constant  Value=G_GNG
  Divide : Product  Inputs=*/
  Gain : Gain  Gain=k_a1
  Gain1 : Gain  Gain=k_a2
  Gain10 : Gain  Gain=1/V_G
  Gain11 : Gain  Gain=0.003*V_G
  Gain12 : Gain  Gain=1/4.5
  Gain14 : Gain  Gain=k_12
  Gain16 : Gain  Gain=S_D
  Gain17 : Gain  Gain=S_E
  Gain2 : Gain  Gain=k_a3
  Gain4 : Gain  Gain=F_01
  Gain7 : Gain  Gain=S_T
  Gain8 : Gain  Gain=-1/(1-1*U_b0/(k_e*V_I*W)*S_E)
  Gain9 : Gain  Gain=E_max-G_GNG
  Integrator : Integrator  InitialCondition=1*U_b0/(k_e*V_I*W)*S_T
  Integrator1 : Integrator  InitialCondition=1*U_b0/(k_e*V_I*W)*S_D
  Integrator2 : Integrator  InitialCondition=U_b0/(k_e*V_I*W)*S_E
  Integrator5 : Integrator  InitialCondition=BG_0*V_G/18
  Integrator6 : Integrator  InitialCondition=S_T*(1*U_b0/(k_e*V_I*W))*(BG_0*V_G/18)/(k_12+S_D*(1*U_b0/(k_e*V_I*W)))
  Product1 : Product
  Product2 : Product
  Product3 : Product
  Saturation : Saturate  UpperLimit=E_max-G_GNG  LowerLimit=0
  Saturation1 : Saturate  UpperLimit=20  LowerLimit=0
  Saturation2 : Saturate  UpperLimit=1  LowerLimit=0
  Sum : Sum  Inputs=|+-
  Sum1 : Sum  Inputs=|+-
  Sum2 : Sum  Inputs=|+-
  basal correction 1 : Gain  Gain=100/(1*U_b0/(k_e*V_I*W)*S_T)
  basal correction 3 : Gain  Gain=100/(1*U_b0/(k_e*V_I*W)*S_E)
  basal correctrion 2 : Gain  Gain=100/(1*U_b0/(k_e*V_I*W)*S_D)
  glucose compartments : Scope  NumInputPorts=2
  glucose fluxes : Scope  NumInputPorts=7
  insulin action : Scope  NumInputPorts=3
  BG : Outport
  wires:
  Sum/1 -> Gain/1
  Gain/1 -> Integrator/1
  Integrator/1 -> [x_1], Sum/2  "transport effect"
  Integrator1/1 -> [x_2], Sum1/2  "disposal effect"
  Gain1/1 -> Integrator1/1
  Sum1/1 -> Gain1/1
  Integrator2/1 -> Sum2/2, [x_3]  "endogeous effect"
  Gain2/1 -> Integrator2/1
  Sum2/1 -> Gain2/1
  I/1 -> Gain7/1, Gain17/1, Gain16/1
  C/1 -> Add Constant/1, Divide/1
  Add Constant/1 -> Divide/2
  Add Constant1/1 -> Gain8/1
  Divide/1 -> Gain9/1
  Gain8/1 -> Product1/1
  Gain9/1 -> Product1/2
  Constant1/1 -> glucose fluxes/3, Add/3  "gluconeogenesis"
  U/1 -> Add/1, glucose fluxes/1  "gut absorption"
  Gain10/1 -> [G], BG/1  "blood glucose"
  [G] -> Add Constant2/1
  Add Constant2/1 -> Gain11/1
  Gain11/1 -> Saturation1/1
  [G] -> Gain12/1
  Integrator5/1 -> [Q_1], glucose compartments/1  "accessible compartment"
  Add/1 -> Integrator5/1
  Gain4/1 -> glucose fluxes/5, Add/5  "insulin independent flux"
  Saturation1/1 -> Add/6, glucose fluxes/6  "renal clearance"
  Integrator6/1 -> glucose compartments/2, [Q_2]  "nonaccessible compartment"
  Add1/1 -> Integrator6/1
  [x_1] -> Product2/1
  [Q_1] -> Product2/2
  Product2/1 -> Add1/2, Add/7, glucose fluxes/7  "glucose distribution flux"
  [Q_2] -> Gain14/1
  Gain14/1 -> glucose fluxes/4, Add1/1, Add/4  "glucose transport flux"
  [Q_2] -> Product3/2
  [x_2] -> Product3/1
  Product3/1 -> Add1/3  "glucose disposal flux"
  [Q_1] -> Gain10/1
  Gain12/1 -> Saturation2/1
  Saturation2/1 -> Gain4/1
  Gain7/1 -> Sum/1
  Gain16/1 -> Sum1/1
  Gain17/1 -> Sum2/1
  basal correctrion 2/1 -> insulin action/2  "glucose disposal"
  basal correction 1/1 -> insulin action/1  "glucose transport"
  basal correction 3/1 -> insulin action/3  "EGP suppression"
  [x_1] -> basal correction 1/1
  [x_2] -> basal correctrion 2/1
  [x_3] -> basal correction 3/1
  Saturation/1 -> glucose fluxes/2, Add/2  "glycogenolysis"
  [x_3] -> Add Constant1/1
  Product1/1 -> Saturation/1

== system SimBG/Patient/Gut Absorption ==
  note: Unit Conversion: [g/min] -> [umol/kg/min]
  note: Glucose mass due to gut absorption, in absorbed compartment
  note: Glucose mass due to gut absorption, in accessible compartment
  CHO : Inport
  Gain : Gain  Gain=1/(t_max_G)
  Gain1 : Gain  Gain=1/(t_max_G)
  Gain2 : Gain  Gain=1/M_g
  Gain3 : Gain  Gain=A_G
  Gain4 : Gain  Gain=10^6/W
  Integrator : Integrator
  Integrator1 : Integrator
  Sum : Sum  Inputs=-+|
  Sum1 : Sum  Inputs=-+|
  U : Outport
  wires:
  Sum/1 -> Integrator/1
  Sum1/1 -> Integrator1/1
  Integrator/1 -> Gain/1
  Gain/1 -> Sum/1, Sum1/2
  Integrator1/1 -> Gain1/1
  Gain3/1 -> Gain2/1
  CHO/1 -> Gain3/1
  Gain4/1 -> U/1
  Gain1/1 -> Gain4/1, Sum1/1
  Gain2/1 -> Sum/2

== system SimBG/Patient/Insulin PK ==
  note: Insulin concentration in plasma
  note: Insulin mass due to exogenous dosing, in serum
  note: Insulin mass due to exogenous dosing, in SC tissue
  UI : Inport
  Gain : Gain  Gain=1/(t_max_I)
  Gain1 : Gain  Gain=1/(t_max_I)
  Gain2 : Gain  Gain=1/(V_I*W)
  Gain3 : Gain  Gain=k_e
  Integrator : Integrator  InitialCondition=U_b0*t_max_I
  Integrator1 : Integrator  InitialCondition=U_b0*t_max_I
  Integrator2 : Integrator  InitialCondition=U_b0/(k_e*V_I*W)
  Sum : Sum  Inputs=-+|
  Sum1 : Sum  Inputs=-+|
  Sum2 : Sum  Inputs=-+|
  I : Outport
  wires:
  Sum/1 -> Integrator/1
  UI/1 -> Sum/2
  Sum1/1 -> Integrator1/1
  Integrator/1 -> Gain/1
  Gain/1 -> Sum/1, Sum1/2
  Integrator1/1 -> Gain1/1
  Gain1/1 -> Gain2/1, Sum1/1
  Integrator2/1 -> Gain3/1, I/1  "Insulin"
  Sum2/1 -> Integrator2/1
  Gain2/1 -> Sum2/2
  Gain3/1 -> Sum2/1

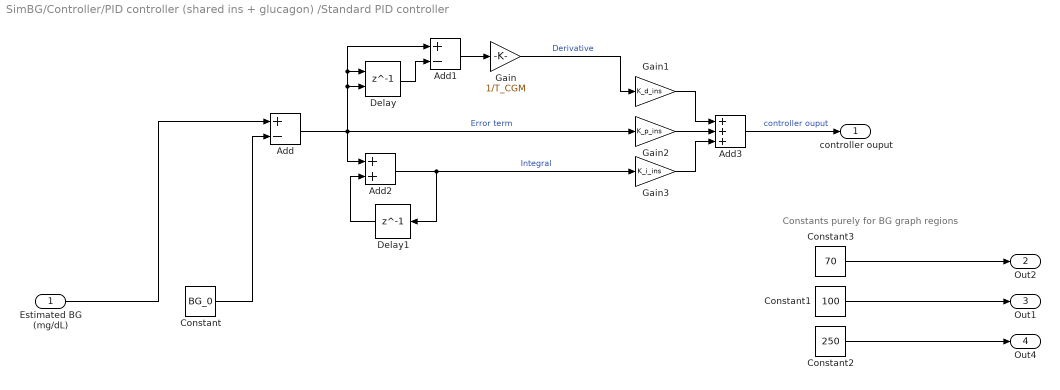
== system SimBG/Controller/PID controller (shared ins + glucagon) /Standard PID controller  ==
  note: Constants purely for BG graph regions
  Estimated BG (mg/dL) : Inport
  Add : Sum  Inputs=+-
  Add1 : Sum  Inputs=+-
  Add2 : Sum
  Add3 : Sum  Inputs=+++
  Constant : Constant  Value=BG_0
  Constant1 : Constant  Value=100
  Constant2 : Constant  Value=250
  Constant3 : Constant  Value=70
  Delay : Delay  DelayLength=1  InitialConditionSource=Input port
      settings: InputPortMap=u0,p4
  Delay1 : Delay  DelayLength=1
  Gain : Gain  Gain=1/T_CGM
  Gain1 : Gain  Gain=K_d_ins
  Gain2 : Gain  Gain=K_p_ins
  Gain3 : Gain  Gain=K_i_ins
  controller ouput : Outport
  Out2 : Outport  Port=2
  Out1 : Outport  Port=3
  Out4 : Outport  Port=4
  wires:
  Delay1/1 -> Add2/2
  Add/1 -> Add2/1, Delay/2, Delay/1, Add1/1, Gain2/1  "Error term"
  Gain/1 -> Gain1/1  "Derivative"
  Delay/1 -> Add1/2
  Add2/1 -> Gain3/1, Delay1/1  "Integral"
  Gain2/1 -> Add3/2
  Constant/1 -> Add/2
  Add1/1 -> Gain/1
  Gain3/1 -> Add3/3
  Constant2/1 -> Out4/1
  Gain1/1 -> Add3/1
  Constant3/1 -> Out2/1
  Add3/1 -> controller ouput/1  "controller ouput"
  Estimated BG (mg/dL)/1 -> Add/1
  Constant1/1 -> Out1/1

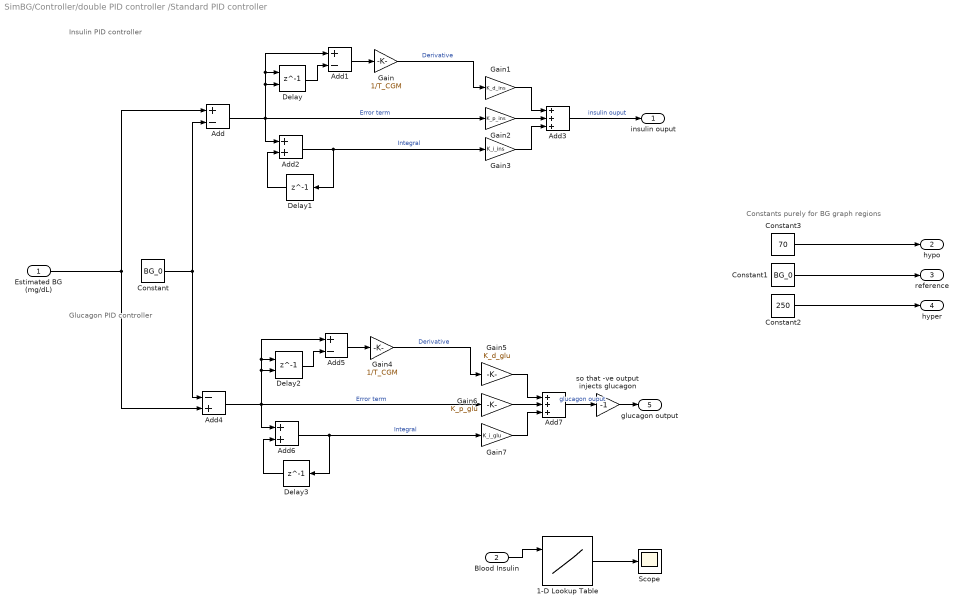
== system SimBG/Controller/double PID controller /Standard PID controller  ==
  note: Glucagon PID controller
  note: Constants purely for BG graph regions
  note: Insulin PID controller
  Estimated BG (mg/dL) : Inport
  Blood Insulin : Inport  Port=2
  1-D Lookup Table : Lookup_n-D  NumberOfTableDimensions=1  BreakpointsForDimension1Source=Input port  BreakpointsForDimension1=[-5:5]  Table=1./(1+exp(-([-5:5])))  InternalRulePriority=Speed  RndMeth=Simplest
      settings: InputPortMap=u0,p5
  Add : Sum  Inputs=+-
  Add1 : Sum  Inputs=+-
  Add2 : Sum
  Add3 : Sum  Inputs=+++
  Add4 : Sum  Inputs=-+
  Add5 : Sum  Inputs=+-
  Add6 : Sum
  Add7 : Sum  Inputs=+++
  Constant : Constant  Value=BG_0
  Constant1 : Constant  Value=BG_0
  Constant2 : Constant  Value=250
  Constant3 : Constant  Value=70
  Delay : Delay  DelayLength=1  InitialConditionSource=Input port
      settings: InputPortMap=u0,p4
  Delay1 : Delay  DelayLength=1
  Delay2 : Delay  DelayLength=1  InitialConditionSource=Input port
      settings: InputPortMap=u0,p4
  Delay3 : Delay  DelayLength=1
  Gain : Gain  Gain=1/T_CGM
  Gain1 : Gain  Gain=K_d_ins
  Gain2 : Gain  Gain=K_p_ins
  Gain3 : Gain  Gain=K_i_ins
  Gain4 : Gain  Gain=1/T_CGM
  Gain5 : Gain  Gain=K_d_glu
  Gain6 : Gain  Gain=K_p_glu
  Gain7 : Gain  Gain=K_i_glu
  Scope : Scope
  so that -ve output injects glucagon : Gain  Gain=-1
  insulin ouput : Outport
  hypo : Outport  Port=2
  reference : Outport  Port=3
  hyper : Outport  Port=4
  glucagon output : Outport  Port=5
  wires:
  Delay1/1 -> Add2/2
  Add/1 -> Add2/1, Delay/2, Delay/1, Add1/1, Gain2/1  "Error term"
  Gain/1 -> Gain1/1  "Derivative"
  Delay/1 -> Add1/2
  Add2/1 -> Gain3/1, Delay1/1  "Integral"
  Gain2/1 -> Add3/2
  Constant/1 -> Add4/1, Add/2
  Add1/1 -> Gain/1
  Gain3/1 -> Add3/3
  Constant1/1 -> reference/1
  Constant2/1 -> hyper/1
  Gain1/1 -> Add3/1
  Constant3/1 -> hypo/1
  Add3/1 -> insulin ouput/1  "insulin ouput"
  Gain6/1 -> Add7/2
  Add4/1 -> Add6/1, Delay2/2, Delay2/1, Add5/1, Gain6/1  "Error term"
  Add7/1 -> so that -ve output injects glucagon/1  "glucagon ouput"
  Gain4/1 -> Gain5/1  "Derivative"
  Delay2/1 -> Add5/2
  Gain7/1 -> Add7/3
  Add5/1 -> Gain4/1
  Add6/1 -> Gain7/1, Delay3/1  "Integral"
  Delay3/1 -> Add6/2
  Gain5/1 -> Add7/1
  Estimated BG (mg/dL)/1 -> Add/1, Add4/2
  so that -ve output injects glucagon/1 -> glucagon output/1
  Blood Insulin/1 -> 1-D Lookup Table/1
  1-D Lookup Table/1 -> Scope/1

== system SimBG/Controller/signal reconstructor/Moving Average ==
  CGM : Inport
  Delay : Delay  DelayLength=1  InitialConditionSource=Input port
      settings: InputPortMap=u0,p4
  Delay1 : Delay  InitialConditionSource=Input port
      settings: InputPortMap=u0,p4
  Gain : Gain  Gain=1/3
  Mux : Mux  Inputs=3
  Scope : Scope  NumInputPorts=2
  Sum of Elements : Sum  Inputs=+
  Out1 : Outport
  wires:
  CGM/1 -> Scope/1, Mux/1, Delay1/2, Delay1/1, Delay/2, Delay/1
  Delay/1 -> Mux/2
  Mux/1 -> Sum of Elements/1
  Sum of Elements/1 -> Gain/1
  Gain/1 -> Scope/2, Out1/1
  Delay1/1 -> Mux/3

== system SimBG/Controller/signal reconstructor/Polynomial ==
  CGM : Inport
  Constant : Constant  Value=0
  evaluator : Subsystem
      settings: PortSchema="{\"entries\":[{\"content\":{\"sides\":[{\"content\":{\"connectorIds\":[\"In1\"]},\"type\":\"ConnectorPlacement.EquallySpacedRectSide\",\"uuid\":\"35f34b66-bfab-428a-939d-8069c2283e72\"},{\"content\":{\"connectorIds\":[\"Out1\"],\"side\":\"RIGHT\"},\"type\":\"ConnectorPlacement.EquallySpacedRectSide\",\"uuid\":\"483b8a40-53bf-45e0-bac5-26b40d77782d\"},{\"content\":{\"connectorIds\":[\"In2\"],\"side\":\"TOP\"},\"type\":\"ConnectorPlacement.EquallySpacedRectSide\",\"uuid\":\"4ce84b89-ca41-4d42-b2ec-9ff5fd075a08\"}]},\"type\":\"ConnectorPlacement.EquallySpacedConnector\",\"uuid\":\"10e137d6-2c4a-4d88-82f6-7acb07ef0bba\"}],\"packageUris\":[\"http://schema.mathworks.com/mf0/Connector/R2020b\"],\"version\":\"1.0\"}"
  poly fitter : Subsystem
  Out1 : Outport
  wires:
  CGM/1 -> poly fitter/1(In1)
  poly fitter/1(Out1) -> evaluator/1(params)
  Constant/1 -> evaluator/2(extrapolation)
  evaluator/1(Out1) -> Out1/1

== system SimBG/Controller/signal reconstructor/Polynomial/evaluator ==
  params : Inport
  extrapolation : Inport  Port=2
  Constant : Constant
  Constant1 : Constant  Value=2
  Constant2 : Constant  Value=3
  Dot Product : DotProduct  OutDataTypeStr=Inherit: Inherit via internal rule
  Mux : Mux
  Power : Math  Operator=pow
  Power1 : Math  Operator=pow
  Out1 : Outport
  wires:
  Constant2/1 -> Power1/2
  Constant1/1 -> Power/2
  params/1 -> Dot Product/1
  Mux/1 -> Dot Product/2
  Dot Product/1 -> Out1/1
  extrapolation/1 -> Power1/1, Power/1, Mux/3
  Constant/1 -> Mux/4
  Power1/1 -> Mux/2
  Power/1 -> Mux/1

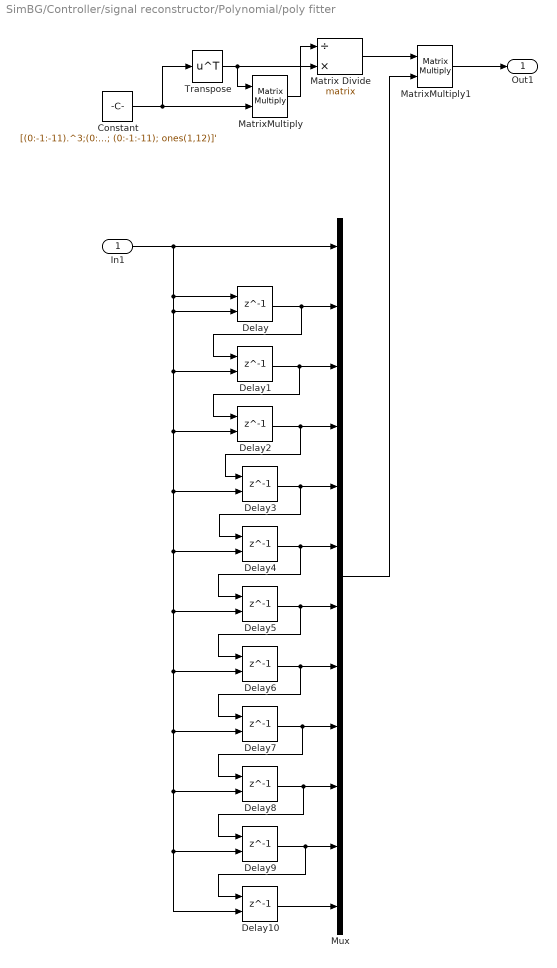
== system SimBG/Controller/signal reconstructor/Polynomial/poly fitter ==
  In1 : Inport
  Constant : Constant  Value=[(0:-1:-11).^3;(0:-1:-11).^2; (0:-1:-11); ones(1,12)]'
  Delay{,1..10} (11 alike) : Delay  DelayLength=1  InitialConditionSource=Input port
      settings: InputPortMap=u0,p4
  Matrix Divide : Product  Inputs=/*  Multiplication=Matrix(*)
  MatrixMultiply : Product  Multiplication=Matrix(*)
  MatrixMultiply1 : Product  Multiplication=Matrix(*)
  Mux : Mux  Inputs=12
  Transpose : Math  Operator=transpose
  Out1 : Outport
  wires:
  In1/1 -> Mux/1, Delay5/2, Delay10/2, Delay9/2, Delay8/2, Delay7/2, Delay6/2, Delay4/2, Delay3/2, Delay2/2, Delay1/2, Delay/2, Delay/1
  Delay/1 -> Delay1/1, Mux/2
  Delay1/1 -> Delay2/1, Mux/3
  Delay2/1 -> Delay3/1, Mux/4
  Delay3/1 -> Delay4/1, Mux/5
  Delay4/1 -> Delay5/1, Mux/6
  Delay5/1 -> Delay6/1, Mux/7
  Delay6/1 -> Delay7/1, Mux/8
  Delay7/1 -> Delay8/1, Mux/9
  Delay8/1 -> Delay9/1, Mux/10
  Delay9/1 -> Delay10/1, Mux/11
  Delay10/1 -> Mux/12
  Constant/1 -> MatrixMultiply/2, Transpose/1
  Transpose/1 -> Matrix Divide/2, MatrixMultiply/1
  MatrixMultiply/1 -> Matrix Divide/1
  Matrix Divide/1 -> MatrixMultiply1/1
  Mux/1 -> MatrixMultiply1/2
  MatrixMultiply1/1 -> Out1/1

== matlab function SimBG/Controller/signal reconstructor/MATLAB Function ==
  data: weight_ih_l0 input; weight_hh_l0 input; bias_ih_l0 input; bias_hh_l0 input; x input; h_next output; h_prev input
function h_next = GRUBlock(weight_ih_l0, weight_hh_l0, bias_ih_l0, bias_hh_l0, x, h_prev)
% GRUBlock implements a GRU cell using PyTorch-style parameters.
%
% Args:
%   x (vector): Input feature at the current timestep.
%   h_prev (vector): Previous hidden state.
%   weight_ih_l0 (matrix): Input-to-hidden weights (3H x input_size).
%   weight_hh_l0 (matrix): Hidden-to-hidden weights (3H x H).
%   bias_ih_l0 (vector): Input-to-hidden biases (3H).
%   bias_hh_l0 (vector): Hidden-to-hidden biases (3H).
%
% Returns:
%   h_next (vector): Updated hidden state.

% Determine hidden size
hidden_size = size(weight_hh_l0, 1) / 3;

% Extract weights for each gate
W_ir = weight_ih_l0(1:hidden_size, :); % Input-to-reset
W_iz = weight_ih_l0(hidden_size+1:2*hidden_size, :); % Input-to-update
W_in = weight_ih_l0(2*hidden_size+1:end, :); % Input-to-candidate

U_r = weight_hh_l0(1:hidden_size, :); % Hidden-to-reset
U_z = weight_hh_l0(hidden_size+1:2*hidden_size, :); % Hidden-to-update
U_n = weight_hh_l0(2*hidden_size+1:end, :); % Hidden-to-candidate

% Extract biases for each gate
b_r = bias_ih_l0(1:hidden_size) + bias_hh_l0(1:hidden_size); % Reset gate bias
b_z = bias_ih_l0(hidden_size+1:2*hidden_size) + bias_hh_l0(hidden_size+1:2*hidden_size); % Update gate bias
b_n = bias_ih_l0(2*hidden_size+1:end) + bias_hh_l0(2*hidden_size+1:end); % Candidate gate bias

% Compute gates
r_t = sigmoid(W_ir * x + U_r * h_prev + b_r); % Reset gate
z_t = sigmoid(W_iz * x + U_z * h_prev + b_z); % Update gate
n_t = tanh(W_in * x + r_t .* (U_n * h_prev) + b_n); % Candidate state

% Compute next hidden state
h_next = (1 - z_t) .* n_t + z_t .* h_prev;
end

% Sigmoid function
function y = sigmoid(x)
    y = 1 ./ (1 + exp(-x));
end

== matlab function SimBG/Controller/MPC controller/MPC Function ==
  data: y input; u output
function u = fcn(y)
% Define system dynamics 
%state space model

Ass = [-3.038*10^-3 -433.12 433.12; 0 -0.012 0; 0 0 -0.017];
Bss = [0 0; 9.27*10^-6 0; 0 2.34*10^-6];

Ts = 5;%sampleing period

A = Ass.*Ts + 1;

n = size(A, 1); % #states = 3 

B = Bss.*Ts;

p = size(B, 2); % #inputs = 2 

% Define cost matrices 

Q = diag([10, 1, 1]); % State cost (glucose more important) 

R = diag([1, 1]); % Control cost (insulin/glucagon effort) 

Qf = Q; % Terminal cost 

% Prediction Horizon 

N = 5; 

% Reference signal 

r = 100; 

%r_vec = repmat([r; r; r], N+1, 1);% Extend reference for the horizon 

% Construct M and C matrices 

M = [eye(n); zeros(N*n, n)];  

C = zeros((N+1)*n, N*p); 

tmp = eye(n);  

for i = 1:N  

rows = i*n + (1:n);  

C(rows,:) = [tmp*B, C(rows-n, 1:end-p)];  

tmp = A * tmp;  

M(rows, :) = tmp;  

end  

% Define Q_bar and R_bar 

Q_bar = kron(eye(N), Q); 

Q_bar = blkdiag(Q_bar, Qf); 

R_bar = kron(eye(N), R);  

% Compute quadratic program matrices 

F = C' * Q_bar * M; % Adjust for reference  

H = C' * Q_bar * C + R_bar;  

G = M' * Q_bar * M;

% Solve QP problem 


% Optimization options 

options = optimoptions('quadprog', 'Algorithm', 'active-set', 'Display', 'off'); 

x0 = [y-r;0;0]; 

X0 = zeros(1,2*N); 


% Solve QP problem with proper argument structure 

u_k = quadprog(H, 2.*x0'*F', [], [], [], [], zeros(1,2*N)', [], X0, options); 

% Extract first control action 

u = u_k(1:p);
%u(1,1) muU/ml
%u(2,1) pg/ml
%align the units
u(1,1) = u(1,1)*10^-3;


y = u;

== matlab function SimBG/Controller/signal reconstructor/MATLAB Function1 ==
  data: h input; y output; W input; b input
function y = FullyConnected(h, W, b)
% FullyConnected computes a dense layer with ReLU activation.
%
% Args:
%   h (vector): Input vector.
%   W (matrix): Weight matrix.
%   b (vector): Bias vector.
%
% Returns:
%   y (vector): Output of the dense layer.

% Compute dense layer output
y = W * h + b;

% Apply ReLU activation
y = max(0, y); % ReLU activation
end

== matlab function SimBG/Controller/signal reconstructor/MATLAB Function2 ==
  data: h input; y output; W input; b input
function y = FullyConnected(h, W, b)
% FullyConnected computes a dense layer with ReLU activation.
%
% Args:
%   h (vector): Input vector.
%   W (matrix): Weight matrix.
%   b (vector): Bias vector.
%
% Returns:
%   y (vector): Output of the dense layer.

% Compute dense layer output
y = reshape(W, 1, []) * h + b;

% Apply ReLU activation
y = max(0, y); % ReLU activation
end

== stateflow chart SimBG/Controller/Controller State Manager/Chart ==
  state init
    timer_on=false;
    CTRL_select=1;
  state controlled
    timer_on=true;
    CTRL_select=1;
  state real_life
    state feed_back
      timer_on=false;
      CTRL_select=feedback_scheme;
    state feed_forward
      timer_on=true;
      CTRL_select=feedforw_scheme;
    (default) -> feed_back
    feed_back -> feed_forward : [Announcement>0]
    feed_forward -> feed_back : [timer>t_ref || ff_exit_flag]
  (default) -> init
  init -> controlled [order 1] : [control_flag]
  init -> real_life [order 2] : [~control_flag]
  data: timer input; t_ref input; ff_exit_flag input; feedback_scheme input; feedforw_scheme input; timer_on output; control_flag input; CTRL_select output; Announcement input
